simulink model "q_9"  (R2020a)
settings: Solver=VariableStepAuto  StartTime=0.0  StopTime=10.0  RelTol=1e-3
values from neighbouring files (symbols this model uses):
  kd = 0    [gain.mat]    (also in gains.mat)
  ki = 1    [gain.mat]    (also in gains.mat = 0)
  kp = 1    [gain.mat]    (also in gains.mat)
settings Model: EnablePacing=on  PacingRate=9  Creator=Admin  LastModifiedBy=Admin

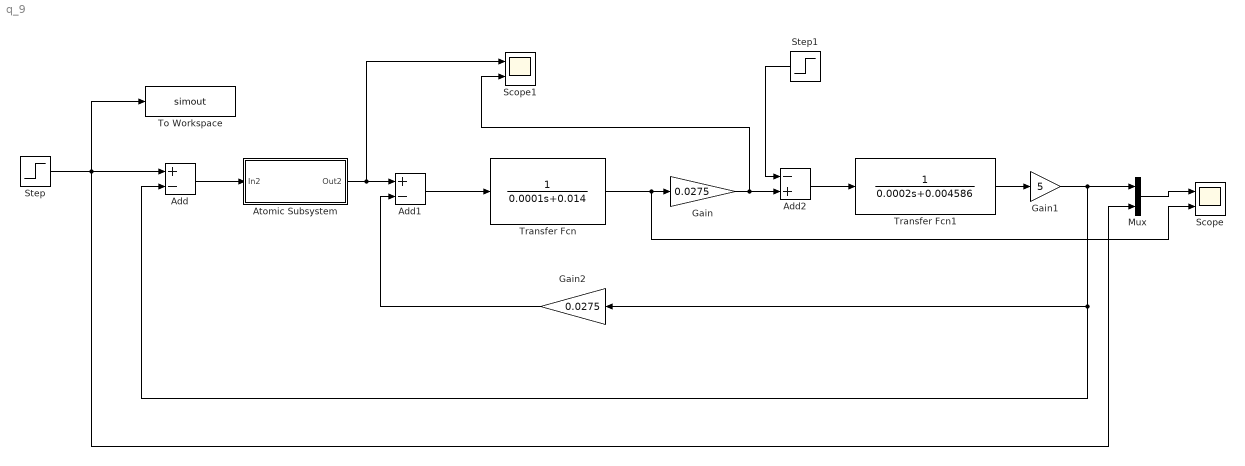
== system q_9 ==
  Add : Sum  Inputs=+-
  Add1 : Sum  Inputs=+-
  Add2 : Sum  Inputs=-+
  Atomic Subsystem : Subsystem  TreatAsAtomicUnit=on
  Gain : Gain  Gain=0.0275
  Gain1 : Gain  Gain=5
  Gain2 : Gain  Gain=0.0275
  Mux : Mux  Inputs=2
  Scope : Scope  NumInputPorts=2
  Scope1 : Scope  NumInputPorts=2
  Step : Step  SampleTime=0
  Step1 : Step  SampleTime=0
  To Workspace : ToWorkspace  VariableName=simout  SaveFormat=Timeseries  SampleTime=-1
  Transfer Fcn : TransferFcn  Denominator=[0.0001 0.014]
  Transfer Fcn1 : TransferFcn  Denominator=[0.0002 0.004586]
  wires:
  Add/1 -> Atomic Subsystem/1(In2)
  Step/1 -> To Workspace/1, Mux/2, Add/1
  Atomic Subsystem/1(Out2) -> Scope1/1, Add1/1
  Add1/1 -> Transfer Fcn/1
  Transfer Fcn/1 -> Scope/2, Gain/1
  Gain/1 -> Scope1/2, Add2/2
  Add2/1 -> Transfer Fcn1/1
  Transfer Fcn1/1 -> Gain1/1
  Gain1/1 -> Gain2/1, Add/2, Mux/1
  Mux/1 -> Scope/1
  Gain2/1 -> Add1/2
  Step1/1 -> Add2/1

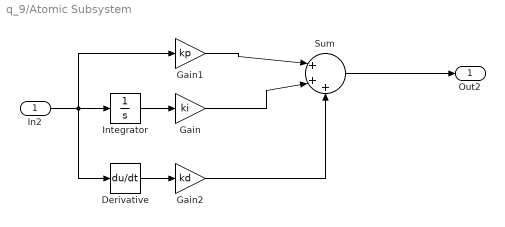
== system q_9/Atomic Subsystem ==
  In2 : Inport
  Derivative : Derivative
  Gain : Gain  Gain=ki
  Gain1 : Gain  Gain=kp
  Gain2 : Gain  Gain=kd
  Integrator : Integrator
  Sum : Sum  Inputs=|+++
  Out2 : Outport
  wires:
  Integrator/1 -> Gain/1
  Derivative/1 -> Gain2/1
  Gain1/1 -> Sum/1
  Gain/1 -> Sum/2
  Gain2/1 -> Sum/3
  Sum/1 -> Out2/1
  In2/1 -> Derivative/1, Gain1/1, Integrator/1
